simulink model "conversor"  (Simulink 5.0)
settings: Solver=ode45  StartTime=0.0  StopTime=10.0  RelTol=1e-3
settings Model: LastModifiedBy=maria  ExtModeTrigMode=oneshot  ExtModeArmWhenConnect=off  LimitDataPoints=off  BooleanDataType=off

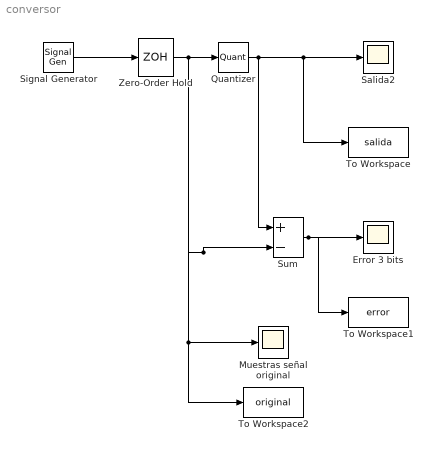
== system conversor ==
  Error 3 bits : Scope
      settings: TimeRange=10
  Muestras señal original : Scope
  Quantizer : Quantizer  QuantizationInterval=10/8
  Salida2 : Scope
  Signal Generator : SignalGenerator  Amplitude=10
  Sum : Sum  Inputs=|+-  SaturateOnIntegerOverflow=on  InputSameDT=on
  To Workspace : ToWorkspace  VariableName=salida  SampleTime=-1  SaveFormat=Array
  To Workspace1 : ToWorkspace  VariableName=error  SampleTime=-1  SaveFormat=Array
  To Workspace2 : ToWorkspace  VariableName=original  SampleTime=-1  SaveFormat=Array
  Zero-Order Hold : ZeroOrderHold  SampleTime=0.01
  wires:
  Signal Generator/1 -> Zero-Order Hold/1
  Quantizer/1 -> Salida2/1, To Workspace/1, Sum/1
  Zero-Order Hold/1 -> Quantizer/1, Sum/2, To Workspace2/1, Muestras señal original/1
  Sum/1 -> To Workspace1/1, Error 3 bits/1
